simulink library "gnc2_lib"  (R2016b)
settings: Solver=VariableStepAuto  StartTime=0.0  StopTime=10.0  RelTol=1e-3
settings Model: Creator=Taylor  LastModifiedBy=taylorreynolds

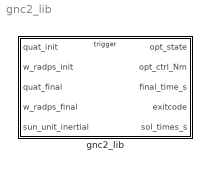
== system gnc2_lib ==
  gnc2_lib : Subsystem

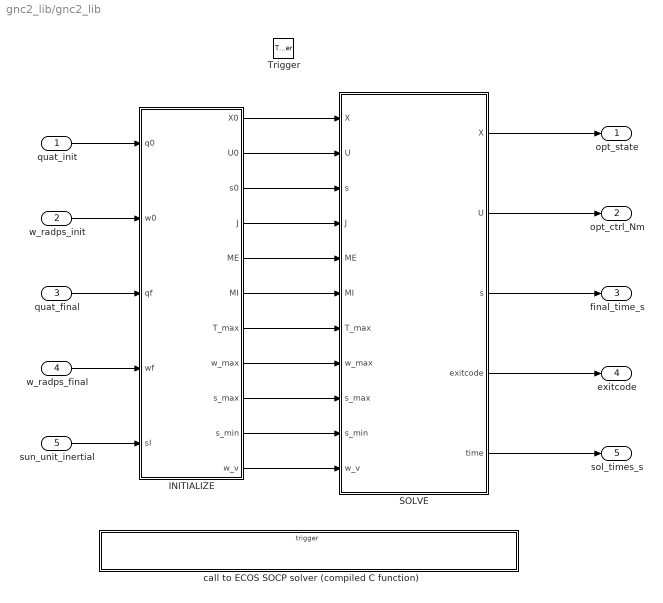
== system gnc2_lib/gnc2_lib ==
  quat_init : Inport
  w_radps_init : Inport  Port=2
  quat_final : Inport  Port=3
  w_radps_final : Inport  Port=4
  sun_unit_inertial : Inport  Port=5
  Trigger : TriggerPort  VariantControl=Variant  StatesWhenEnabling=reset  ZeroCross=off  InitialTriggerSignalState=zero  PortDimensions=1
  INITIALIZE : MATLAB Function  TreatAsAtomicUnit=on
  SOLVE : MATLAB Function  TreatAsAtomicUnit=on
  call to ECOS SOCP solver (compiled C function) : Subsystem  TreatAsAtomicUnit=on
  opt_state : Outport
  opt_ctrl_Nm : Outport  Port=2
  final_time_s : Outport  Port=3
  exitcode : Outport  Port=4
  sol_times_s : Outport  Port=5
  wires:
  sun_unit_inertial/1 -> INITIALIZE/5(sI)
  w_radps_final/1 -> INITIALIZE/4(wf)
  quat_final/1 -> INITIALIZE/3(qf)
  w_radps_init/1 -> INITIALIZE/2(w0)
  quat_init/1 -> INITIALIZE/1(q0)
  INITIALIZE/1(X0) -> SOLVE/1("X ")
  INITIALIZE/11(w_v) -> SOLVE/11(w_v)
  INITIALIZE/2(U0) -> SOLVE/2("U ")
  INITIALIZE/3(s0) -> SOLVE/3("s ")
  INITIALIZE/4(J) -> SOLVE/4(J)
  INITIALIZE/5(ME) -> SOLVE/5(ME)
  INITIALIZE/6(MI) -> SOLVE/6(MI)
  INITIALIZE/7(T_max) -> SOLVE/7(T_max)
  INITIALIZE/8(w_max) -> SOLVE/8(w_max)
  INITIALIZE/9(s_max) -> SOLVE/9(s_max)
  INITIALIZE/10(s_min) -> SOLVE/10(s_min)
  SOLVE/1(X) -> opt_state/1
  SOLVE/2(U) -> opt_ctrl_Nm/1
  SOLVE/3(s) -> final_time_s/1
  SOLVE/4(exitcode) -> exitcode/1
  SOLVE/5(time) -> sol_times_s/1

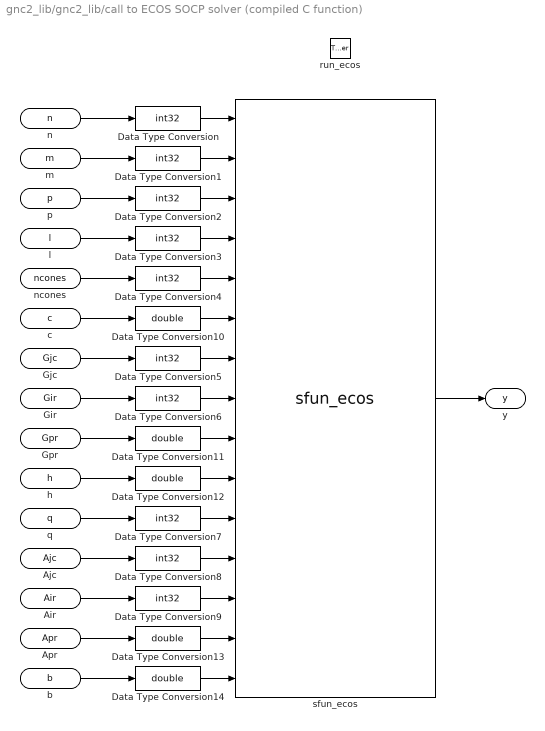
== system gnc2_lib/gnc2_lib/call to ECOS SOCP solver (compiled C function) ==
  run_ecos : TriggerPort  TriggerType=function-call  IsSimulinkFunction=on  FunctionName=run_ecos  VariantControl=(inherit)
  Data Type Conversion{,1..9} (10 alike) : DataTypeConversion  OutDataTypeStr=int32
  Data Type Conversion{10..14} (5 alike) : DataTypeConversion  OutDataTypeStr=double
  sfun_ecos : S-Function  FunctionName=sfun_ecos  SFunctionDeploymentMode=off  EnableBusSupport=off  mask(Legacy Function){}
      mask help:
      | This block allows you to call the legacy functions specified by the following Legacy Code Tool definition:
      | def.SFunctionName = 'sfun_ecos';
      | def.OutputFcnSpec = 'solve_simple_optimization(int32 p1,int32 p2,int32 p3,int32 p4,int32 p5,double p6[18],int32 p7[19],int32 p8[57],double u1[57],double u2[38],int32 p9[6],int32 p10[19],int32 p11[16],double u3[16],double u4[6],solution y1[1])';
      | def.HeaderFiles = {'ecos.h', 'matlab_header.h'};
      | def.SourceFiles = {'main.c', 'cone.c', 'ctrlc.c', 'ecos.c', 'equil.c', 'expcone.c', 'kkt.c', 'preproc.c', 'spla.c', 'splamm.c', 'timer.c', 'wright_omega.c', 'ldl.c', 'amd_1.c', 'amd_2.c', 'amd_aat.c', 'amd_control.c', 'amd_defaults.c', 'amd_dump.c', 'amd_global.c', 'amd_info.c', 'amd_order.c', 'amd_post_tree.c', 'amd_postorder.c', 'amd_preprocess.c', 'amd_valid.c'};
      | def.IncPaths = {'./ecos/include', './ecos/external/ldl/include', './ecos/external/amd/include', './ecos/external/SuiteSparse_config'};
      | def.SrcPaths = {'./ecos/src', './ecos/external/ldl/src', './ecos/external/amd/src'};
      mask Help: <p>This block was generated automatically by the Legacy Code Tool. For detailed help on this tool, call<a href="matlab:legacy_code('help')"> legacy_code('help')</a>.</p>
      mask DialogControl DescGroupVar Prompt: Convex optimization
      mask DialogControl DescTextVar Prompt: <b>Mathematical Description of SOACer</b><br><br>  Computes one solve step of the optimal attitude reorientation problem by solving a minimum-time constrained attitute control problem via convex optimization. Formulation: <br> <br> min c'*z<br>subject to<br>A*z=b<br>G*z&lt;=_K h <br> <br> Where &lt;=_K denotes a generalized inequality with respect to the cone K, i.e. the vector h-G*z belongs to the cone K. The cone K may be an n-dimensional positive orthant (R_+^n, which simply means G*z &lt;=h is the usual inequality) or a second-order Q^n defined as: <br> <br> Q^n = {(t(z),x(z)) in R x R^{n-1} | t(z) &lt;= ||x(z)||_2} <br> <br> For the latter case, h-G*z defines then the (t,x) in R^n vector. The case of exponential cones, which ECOS can handle, does not appear in the attitude control problem problem and is not considered here.<br><br> <b>ECOS C API</b><br><br> n : Number of primal variables<br> m : Number of generalized inequality constraints, i.e. dimension 1 of matrix G and length of vector h<br> p : Number of equality constraints, i.e. dimension 1 of matrix A and length of vector b<br> l : Dimension of the positive orthan R_+^l (number of usual inequality constraints)<br> ncones : Number of second-order cones<br> q : Array of length ncones; q[i] defines the dimension of the cone i<br> Gpr, Gjc, Gir : Arrays of matrix G in column compressed storage (CCS)<br> Apr, Ajc, Air : Arrays of matrix A in column compressed storage (CCS)<br> c : Array of length n (cost)<br> h : Array of length m (RHS of generalized inequality constraints)<br> b : Array of length p (RHS of equality constraints)<br>
      mask Display:
      | %%% Input port labels
      | port_label('input',1,'n');
      | port_label('input',2,'m');
      | port_label('input',3,'p');
      | port_label('input',4,'l');
      | port_label('input',5,'ncones');
      | port_label('input',6,'c');
      | port_label('input',7,'Gjc');
      | port_label('input',8,'Gir');
      | port_label('input',9,'Gpr');
      | port_label('input',10,'h');
      | port_label('input',11,'q');
      | port_label('input',12,'Ajc');
      | port_label('input',13,'Air');
      | port_label('input',14,'Apr');
      | port_label('input',15,'b');
      | %%% Outputs port labels
      | port_label('output',1,'optimal_solution');
  n : ArgIn  DisableCoverage=on  ArgumentName=n
  m : ArgIn  DisableCoverage=on  Port=2  ArgumentName=m
  p : ArgIn  DisableCoverage=on  Port=3  ArgumentName=p
  l : ArgIn  DisableCoverage=on  Port=4  ArgumentName=l
  ncones : ArgIn  DisableCoverage=on  Port=5  ArgumentName=ncones
  c : ArgIn  DisableCoverage=on  Port=6  PortDimensions=soac_params.c_size  ArgumentName=c
  Gjc : ArgIn  DisableCoverage=on  Port=7  PortDimensions=soac_params.Gjc_size  ArgumentName=Gjc
  Gir : ArgIn  DisableCoverage=on  Port=8  PortDimensions=soac_params.Gir_size  ArgumentName=Gir
  Gpr : ArgIn  DisableCoverage=on  Port=9  PortDimensions=soac_params.Gpr_size  ArgumentName=Gpr
  h : ArgIn  DisableCoverage=on  Port=10  PortDimensions=soac_params.h_size  ArgumentName=h
  q : ArgIn  DisableCoverage=on  Port=11  PortDimensions=soac_params.q_size  ArgumentName=q
  Ajc : ArgIn  DisableCoverage=on  Port=12  PortDimensions=soac_params.Ajc_size  ArgumentName=Ajc
  Air : ArgIn  DisableCoverage=on  Port=13  PortDimensions=soac_params.Air_size  ArgumentName=Air
  Apr : ArgIn  DisableCoverage=on  Port=14  PortDimensions=soac_params.Apr_size  ArgumentName=Apr
  b : ArgIn  DisableCoverage=on  Port=15  PortDimensions=soac_params.b_size  ArgumentName=b
  y : ArgOut  DisableCoverage=on  PortDimensions=soac_params.y_size  ArgumentName=y
  wires:
  sfun_ecos/1 -> y/1
  n/1 -> Data Type Conversion/1
  m/1 -> Data Type Conversion1/1
  p/1 -> Data Type Conversion2/1
  l/1 -> Data Type Conversion3/1
  ncones/1 -> Data Type Conversion4/1
  Ajc/1 -> Data Type Conversion8/1
  Air/1 -> Data Type Conversion9/1
  Apr/1 -> Data Type Conversion13/1
  b/1 -> Data Type Conversion14/1
  c/1 -> Data Type Conversion10/1
  Gjc/1 -> Data Type Conversion5/1
  Gir/1 -> Data Type Conversion6/1
  Gpr/1 -> Data Type Conversion11/1
  h/1 -> Data Type Conversion12/1
  q/1 -> Data Type Conversion7/1
  Data Type Conversion/1 -> sfun_ecos/1
  Data Type Conversion1/1 -> sfun_ecos/2
  Data Type Conversion2/1 -> sfun_ecos/3
  Data Type Conversion3/1 -> sfun_ecos/4
  Data Type Conversion4/1 -> sfun_ecos/5
  Data Type Conversion5/1 -> sfun_ecos/7
  Data Type Conversion6/1 -> sfun_ecos/8
  Data Type Conversion7/1 -> sfun_ecos/11
  Data Type Conversion8/1 -> sfun_ecos/12
  Data Type Conversion9/1 -> sfun_ecos/13
  Data Type Conversion10/1 -> sfun_ecos/6
  Data Type Conversion11/1 -> sfun_ecos/9
  Data Type Conversion12/1 -> sfun_ecos/10
  Data Type Conversion13/1 -> sfun_ecos/14
  Data Type Conversion14/1 -> sfun_ecos/15

== matlab function gnc2_lib/INITIALIZE ==
  data: q0 input; w0 input; qf input; wf input; sI input; X0 output; U0 output; s0 output; J output; ME output; MI output; T_max output; w_max output; s_max output; s_min output; w_v output
function [X0,U0,s0,J,ME,MI,T_max,w_max,s_max,s_min,w_v] = init_SOACer(q0,w0,qf,wf,sI)
%INIT_SOACER    
%
% SOACer's init function.
%
% T. Reynolds -- RAIN Lab

%#codegen

% Constraints
cB       = [ 0.0; 0.0; -1.0 ]; % Camera boresight vector
amax     = deg2rad(60);        % FOV cone size
M        = [ sI*cB'+cB*sI'-(sI'*cB)*eye(3)   skew(sI)*cB;
             (skew(sI)*cB)'                  sI'*cB ] - cos(amax)*eye(4);
Mt       = M + 2*eye(4);    % M_tilde
% compute matrix square root. Cannot use ME = sqrtm(Mt) since complex
% values are returned, and these are turned off for code generation
[V,D] = schur(Mt);
for k = 1:4
    D(k,k) = realsqrt(D(k,k));
end
ME  = V*D*V';           % Exclusion constraint matrix
MI  = zeros(size(ME));  % Inclusion constraint matrix
s_min   = 0.5;  % min allowable time
s_max   = 15;   % max allowable time

% Controller parameters
N       = 10;   % number of time nodes
Nx      = 7;    % number of states
Nu      = 3;    % number of controls

% spacecraft inertia matrix
J       = [ 0.0338    -4.884e-05 -7.393e-05;
            -4.884e-05  0.0346     7.124e-06;
            -7.393e-05  7.124e-06  0.0075 ]; % kg m2
T_max   = 1e-3; % 1mNm
w_max   = 0.3;  % rad/s
w_v     = 1e2;  % virtual control weight

% Initial trajectory
x0  = zeros(7,N);
u0  = zeros(3,N);
s0  = 2.0467; 
tau = linspace(0,1,N);
[qb,flag] = Q_SLERP(q0,qf);
if ( flag == 0 )
    for k = 1:N
        wk = zeros(3,1);
        for i = 1:3
           wk(i) = interp1([0 1],[w0(i) wf(i)],tau(k),'linear');
        end
        x0(:,k)   = [ qb(:,k); wk ];
        u0(:,k)     = zeros(3,1);
    end
end

% Initial state and control guess
X0   = reshape(x0,Nx*N,1);
U0   = reshape(u0,Nu*N,1);

end

function [qt,FLAG] = Q_SLERP( q0,q1 )
%Q_SLERP 
%
% Q_SLERP(q0,q1,tspan) Uses Spherical Linear intERPolation to 
% interpolate between two quaternions given the time space tspan. 
% Both q0 and q1 must be quaternions.
%
% T.Reynolds -- RAIN Lab.
%#codegen

N    = 10;
FLAG = int8(0);

if ( length(q0)~=4 || length(q1)~=4 )
   FLAG = int8(1);
   qt   = repmat([1.0;0.0;0.0;0.0],1,N);
   return;
end

% Reshape inputs to be column vectors
q0  = reshape(q0, 4, 1);
q1  = reshape(q1, 4 ,1);

% Find angle between inputs
ang = acos(dot(q0,q1));
if ( ang > pi )
    FLAG = int8(2);
    qt   = repmat([1.0;0.0;0.0;0.0],1,N);
    return;
end

sang = sin(ang);
qt   = zeros(4,N);
for k = 1:N
    t       = (k-1)/(N-1);
    qt(:,k) = (sin((1 - t)*ang)/sang).*q0 + (sin(t*ang)/sang).*q1;
end

end

== matlab function gnc2_lib/SOLVE ==
  data: X input; U input; s input; J input; ME input; MI input; T_max input; w_max input; s_max input; s_min input; w_v input; X output; soac_params parameter; U output; s output; exitcode output; time output
function [X,U,s,exitcode,time] = solve_SOACer(X,U,s,J,ME,MI,T_max,w_max,...
                        s_max,s_min,w_v,soac_params)                  
%                         c_size, Air_size, Ajc_size, Apr_size, b_size, ...
%                         Gir_size, Gjc_size, Gpr_size, h_size, q_size)
%SOLVE_STEP     
%
% SOACer's main function that solves the problem fully.
%
% T. Reynolds -- RAIN Lab

%#codegen

% Set problem sizes
N = 10;         % number of time nodes
iter_max = 10;  % maximum global iterations
c_size   = soac_params.c_size;
b_size   = soac_params.b_size;
h_size   = soac_params.h_size;
q_size   = soac_params.q_size;
Air_size = soac_params.Air_size;
Ajc_size = soac_params.Ajc_size;
Apr_size = soac_params.Apr_size;
Gir_size = soac_params.Gir_size;
Gjc_size = soac_params.Gjc_size;
Gpr_size = soac_params.Gpr_size;

n = c_size;     % primal variables
m = h_size;     % number of inequality constraints
p = b_size;     % number of equality constraints
l = h_size;     % WITH NO SOCs (otherwise small than h_size)

ncones   = 0;   % number of second order cones
q        = 0;   % dimension of the ith cone
exitcode = zeros(iter_max+1,1);
time     = zeros(iter_max,1);

% Initial and final conditions stored in initial guess X
xi = X(1:7);
xf = X(7*(N-1)+1:7*N);

for k = 1:iter_max
    
    % discretize
    [EH,BE,ES,AR] = foh(X,U,s,N,J);
    
    % parse for ECOS
    [c,G,h,A,b] = parse_ecos(xi,xf,EH,BE,ES,AR,N,...
                                        ME,MI,T_max,w_max,s_max,s_min,w_v);
    
    % Put A and G in compressed column storage
    [Air,Ajc,Apr] = convert_to_CCS(A,Air_size,Apr_size);
    [Gir,Gjc,Gpr] = convert_to_CCS(G,Gir_size,Gpr_size);
    
    % pad with zeros as needed
    Air = [Air; zeros(Air_size-numel(Air),1)];
    Ajc = [Ajc; zeros(Ajc_size-numel(Ajc),1)];
    Apr = [Apr; zeros(Apr_size-numel(Apr),1)];
    Gir = [Gir; zeros(Gir_size-numel(Gir),1)];
    Gjc = [Gjc; zeros(Gjc_size-numel(Gjc),1)];
    Gpr = [Gpr; zeros(Gpr_size-numel(Gpr),1)];
       
    % Call to ECOS
    y = run_ecos(n,m,p,l,ncones,c(1:c_size),...
                    Gjc(1:Gjc_size),Gir(1:Gir_size),Gpr(1:Gpr_size),...
                    h(1:h_size),q(1:q_size),...
                    Ajc(1:Ajc_size),Air(1:Air_size),Apr(1:Apr_size),...
                    b(1:b_size));
    
    % Check convergence & update solution
    diff        = norm(X - y(1:70),1); % difference in state vector
    X           = y(1:70);
    U           = y(71:100);
    s           = y(101);
    V           = y(102:171);
    exitcode(k) = y(c_size+1);
    time(k)     = y(c_size+2);
    % if one of the exitcodes indicates failue, the final
    % entry in exitcode is set to -1 to indicate this, and the
    % solution should not be used
    if (exitcode(k) ~= 0)
        exitcode(iter_max+1) = -1;
    end
    
    if ( (norm(V,1) < 1e-5) && (diff < 1e-5) )
        % exit for loop since we think we've converged
        break;
    end
            
end

% Sanity checks on the solution if we hit the max iterations
if (k==iter_max) % hit max global iterations
    if (exitcode(iter_max+1) ~= -1 )
        if (norm(V,1) > 1e-5)
            exitcode(iter_max+1) = 3; % does not clash with ECOS exitcodes
        elseif (diff>1e-5)
            exitcode(iter_max+1) = 4;
        end
    end
end

end

%%%%%%%%%%%%%%%%%%%%%%%%%%%%%%%%%%%%%%%%%%%%%%%%%%%%%%%%%%%%%%%%%%%%%%%%%%%
%%%%%%%%%%%%%%%%%%%%%%%%%%%% SUPPORT FUNCTIONS %%%%%%%%%%%%%%%%%%%%%%%%%%%%
%%%%%%%%%%%%%%%%%%%%%%%%%%%%%%%%%%%%%%%%%%%%%%%%%%%%%%%%%%%%%%%%%%%%%%%%%%%

function [ EH,BE,ES,AR ] = foh( X,U,s,N,J )
%FOH   first order hold discretization
%
% FOH(X,U,s,N,J) Computes the matrices (A,B,S,Z) to numerically discretize 
% a problem instance of SOAC about the most recent trajectory 
% stored in X and U. Assumes a linear interpolation of the torque 
% between control nodes, of which there are N.
%
% These matrices give the first order Taylor series of the dynamics
% at the N time nodes dictated and correspond to a discrete time
% LTV system approximating the nonlinear dynamics.
%
% Inputs: 
%   - X (N*Nx by 1) current state at each discrete node
%   - U (N*Nu by 1) current control at each discrete node
%   - s (1 by 1) current final time
%   - N (1 by 1) number of discrete time nodes
%   - J (3 by 3) spacecraft inertia matrix
% Outputs: 
%   - EH (N*Nx by N*Nx)
%   - BE (N*Nu by N*Nu)
%   - ES (N*Nx by 1)
%   - ZE (N*Nx by 1)
%
% T. Reynolds -- RAIN Lab

len     = N-1;              % number of transition matrices
tau     = linspace(0,1,N);  % normalized time
Nsub    = 10;               % number of sub-interval points

% Set sizes for each discrete matrix
EH          = zeros(7*(len+1),7*(len+1));
EH(1:7,1:7) = eye(7);
BE          = zeros(7*(len+1),3*(len+1));
ES          = zeros(7*(len+1),1);
AR          = zeros(7*(len+1),1);

% Initial conditions
A0  = eye(7);
B0p = zeros(21,1);
B0m = zeros(21,1);
S0  = zeros(7,1);
R0  = zeros(7,1);

for k = 1:len
    
    % (re)define initial condition for integration
    xF = X(7*(k-1)+(1:7));
    P0 = [xF(:); A0(:); B0p(:); B0m(:); S0(:); R0(:)];
    
    um = U(3*(k-1)+(1:3));
    up = U(3*k+(1:3));
    u  = [reshape(um,3,1) reshape(up,3,1)];
    tspan = linspace(tau(k), tau(k+1), N);
    
    for k_ = 1:Nsub-1
        
        tk      = tspan(k_);
        tkp1    = tspan(k_+1);
        h       = tkp1-tk;
        
        k1 = deriv(tk    ,P0       ,u,tspan,s,J);
        k2 = deriv(tk+h/2,P0+h/2*k1,u,tspan,s,J);
        k3 = deriv(tk+h/2,P0+h/2*k2,u,tspan,s,J);
        k4 = deriv(tk+h  ,P0+h*k3  ,u,tspan,s,J);
        
        P0 = (P0+h/6*(k1+2*k2+2*k3+k4));
    end
    
    AF  = P0(8:56);
    BFp = P0(57:77);
    BFm = P0(78:98);
    SF  = P0(99:105);
    RF  = P0(106:end);
    
    % Reshape to matrices
    Ad  = reshape(AF,7,7);
    Bdp = Ad*reshape(BFp,7,3);
    Bdm = Ad*reshape(BFm,7,3);
    Sd  = Ad*reshape(SF,7,1);
    Rd  = Ad*reshape(RF,7,1);
    
    % Fill up matrices
    EH(7*k+(1:7),7*(k-1)+(1:7)) = Ad;
    BE(7*k+(1:7),3*(k-1)+(1:3)) = Bdm;
    BE(7*k+(1:7),3*k+(1:3))     = Bdp;
    ES(7*k+(1:7))               = Sd;
    AR(7*k+(1:7))               = Rd;
    
end


end

function DX = deriv(t,X,u,tspan,s,J)

    x   = X(1:7); % Nx = 7
    
    [f,A,Bp,Bm,Z] = get_f_vals(t,x,u,tspan,J);
    
    Phi = reshape(X(8:56),size(A));
       
    xdot        = s*f;
    Phi_dot     = (s*A)*Phi;
    Bdp_dot     = Phi\(s*Bp);
    Bdm_dot     = Phi\(s*Bm);
    Sd_dot      = Phi\f;
    Zd_dot      = Phi\(s*Z);
    
    DX      = [ xdot(:); Phi_dot(:); Bdp_dot(:);...
                Bdm_dot(:); Sd_dot(:); Zd_dot(:)];
end

function [f,A,Bp,Bm,Z] = get_f_vals(t,x,u,tspan,J)
    
    tkm     = tspan(1);
    tkp     = tspan(end);     
    lam_km  = (tkp - t)/(tkp - tkm);
    lam_kp  = (t - tkm)/(tkp - tkm);
    
    % Interpolate u
    u_tau = lam_km .* u(:,1) + lam_kp .* u(:,2);

    % compute jacobian matrices
    [A,B,f] = Q_linearize(t,x,u_tau,J);
    
    Bp  = lam_kp*B;
    Bm  = lam_km*B;
    
    % compute z
    Z   = - A*x - B*u_tau;
                           
end

function [ A,B,f ] = Q_linearize( t,x,u,J )
%Q_LINEARIZE    Linearize the attitude dynamics
%
% Q_linearize(t,x,u,P) returns the discrete representation of the
% quaternion-based attitude dynamics at the point (x,u) and time t. The
% struct P must contain at least an entry called 'inertia'.
%
% T. Reynolds -- RAIN Lab.

% States
q   = x(1:4)./norm(x(1:4));
q0  = q(1);
qv  = q(2:4);
w   = x(5:7);

% Partials
dfq_dq  = 0.5 * [ 0 -w'; w -skew(w) ];
dfq_dw  = 0.5 * [ -qv'; skew(qv)+q0*eye(3) ];
dfw_dq  = zeros(3,4);
dfw_dw  = -J\( skew(w)*J - skew(J*w) );
dfq_du  = zeros(4,3);
dfw_du  = inv(J);

% Kinematics & Dynamics
fq  = 0.5 * [ -qv'; skew(qv)+q0*eye(3) ] * w;
fw  = J\(u - skew(w)*J*w); % CHANGE THIS TO INCLUDE WHEEL MOMENTUM?

% Outputs
f  = [ fq; fw ];
A  = [ dfq_dq dfq_dw; dfw_dq dfw_dw ];
B  = [ dfq_du; dfw_du ];

end

function [c,G,h,A,b] = parse_ecos(xi,xf,EH,BE,ES,AR,N,...
                                    ME,MI,T_max,w_max,s_max,s_min,w_v)

u_max = T_max .* ones(N*3,1);
w_max = w_max .* ones(N*3,1);

% Hx  = [ eye(N*Nx) zeros(N*Nx,N*(Nu+2*Nx)+1) ];
Hw  = [ kron(eye(N),[zeros(3,4) eye(3)]) zeros(3*N,N*(3+2*7)+1) ];
Hu  = [ zeros(N*3,N*7) eye(N*3) zeros(N*3,2*N*7+1) ];
Hv  = [ zeros(N*7) zeros(N*7,N*3) ...
        zeros(N*7,1) eye(N*7) zeros(N*7,N*7) ];
Hs  = [ zeros(1,N*(7+3)) 1 zeros(1,2*N*7) ];
Hev = [ zeros(N*7,N*(2*7+3)+1) eye(N*7) ];

z_xNu = zeros(7,N*3);
z_xNx = zeros(7,N*7);

% Cost function
c   = [ zeros(N*(7+3),1); 1; zeros(N*7,1); w_v*ones(N*7,1) ];
% Equality constraints
A   = [ eye(7) repmat(zeros(7),1,N-1) z_xNu zeros(7,1) z_xNx z_xNx;
        EH-eye(size(EH)) BE ES eye(7*N) zeros(N*7,N*7);
        repmat(zeros(7),1,N-1) eye(7) z_xNu zeros(7,1) z_xNx z_xNx ];
b   = [xi; -AR; xf];
% Inequality constraints
Glin    = [ Hw; -Hw; Hu; -Hu; Hs; -Hs; Hv-Hev; -Hv-Hev ];
% Gquad   = [ ];
G       = Glin;
% G       = sparse([ Glin; Gquad ]);
hlin    = [ w_max; w_max; ...               
            u_max; u_max; ...               
            s_max; -s_min; ...
            zeros(N*7,1); zeros(N*7,1) ];
% hquad   = [ ];
h   = hlin;
% h       = [ hlin; hquad ];

end

function [Mir,Mjc,Mpr] = convert_to_CCS(Mf,Mir_size,Mpr_size)
%     [Mir,~,Mpr] = find(Mf);
    [Mir,Mpr] = my_find(Mf,Mir_size,Mpr_size);
    Mir = Mir-1; % zero-based row indexing
    Mjc = zeros(size(Mf,2)+1,1);
    for col = 2:size(Mf,2)
        Mjc(col) = Mjc(col-1)+nnz(Mf(:,col-1));
    end
    Mjc(end) = Mir_size;
end

function [Mir,Mpr] = my_find(M,Mir_size,Mpr_size)
    Mir = zeros(Mir_size,1);
    Mpr = zeros(Mpr_size,1);
    [n,m] = size(M);
    k = 1;
    for j = 1:m
        for i = 1:n
            if (M(i,j) ~= 0)
                Mir(k) = i;
                Mpr(k) = M(i,j);
                k = k+1;
            end
        end
    end
end
